simulink library "tvd"  (Simulink 8.1)
settings: Solver=ode1  StartTime=0.0  StopTime=Inf  FixedStep=0.001  RelTol=1e-3
PostLoadFcn:
  | , if any(exist('dsrtsu_mdlpostloadfcn', 'file') == [2, 3, 6]), try dsrtsu_mdlpostloadfcn('Execute', bdroot); catch fprintf('Error in PostLoadFcn (dsrtsu_mdlpostloadfcn) for model "%s":\n %s\n', bdroot, lasterr); end, end,
undefined symbols (not defined in the file or in its folder): C_TICK_TIME_S, KACC_MCLongAccelRollAvgInterval_s
libraries: hcu_lib x1
settings Model: DSRTSU_INTERNAL_RTI_VER=450  DSRTSU_INTERNAL_RTI_TYPE=rti1401  RTICANMMDATA=struct('GeneralSetupData',struct('modelroot','D:\Projects\ELN150201\Repositories\Taiwan\trunk\AdasDragon\software\sw_development\arch\app\acc','generalsettings',struct('filesettings',struct('destfolder',struct('Name','RTICANMM_FILES','Check',1),'buildfolder',struct('Name','.','Check',1),'AbsDestfolder',struct('Name','D:\Projects\ELN150201\Repositories\Taiwan\trunk\AdasDragon\software\sw_development\arch\app\acc\RTICANMM_FILES'),'AbsBuildfolder',struct('Name','D:\Projects\ELN150201\Repositories\Taiwan\trunk\AdasDragon\software\sw_development\arch\app\acc'))),'options',struct('addpaths',1,'rmpaths',1,'addtrcexclusion',logical(1),'cannavigator',struct('checkmonitoring',0),'show_usrtrc',0,'use_usrtrc',0),'advanced',struct('options',[1 1 1 1 1 1 1 1 1 1 1 1 1 1 1 1 1 1 1 1 1 1 1 1 1 1 1 1 1 1 1 1 1 1 1 1 1 1 1 1 1 1 1 1 1 1 1 1 1 1 1 1 1 1 1 1 1 1 1 1 1 1 1 1 1 1 1 1 1 1 1 1 1 1 1 1 1 1 1 1 1 1 1 1 1 1 1 1 1 1 1 1 1 1 1 1 1 1 1 1]),'MPSetup',{{}},'modelname','Copy_of_scc','block','Copy_of_scc'))  DSRTSU_INTERNAL_RTIFPGA=40  Creator=AT015411  LastModifiedBy=AT015086

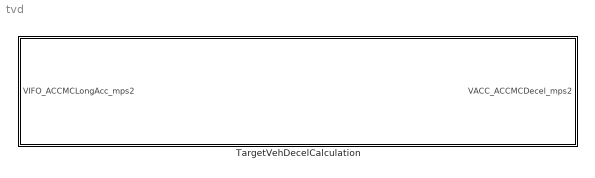
== system tvd ==
  TargetVehDecelCalculation : Subsystem

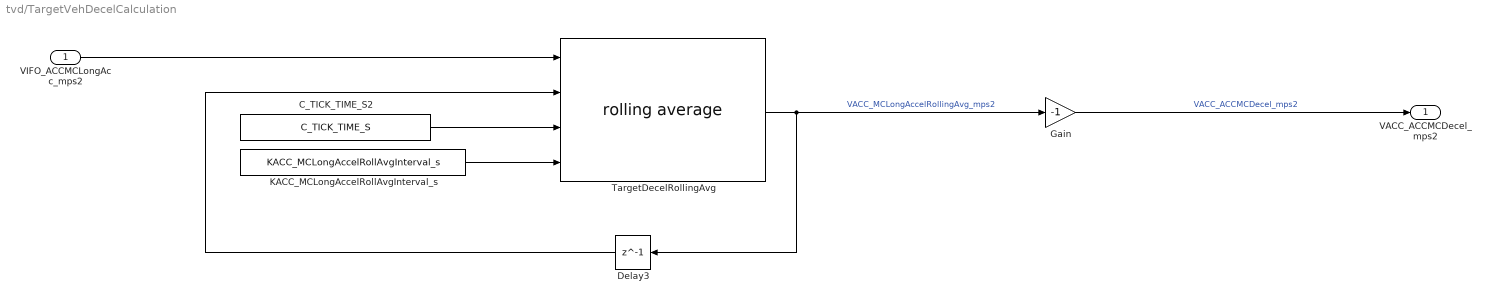
== system tvd/TargetVehDecelCalculation ==
  VIFO_ACCMCLongAcc_mps2 : Inport
  C_TICK_TIME_S2 : Constant  Value=C_TICK_TIME_S
  Delay3 : Delay  DelayLength=1
  Gain : Gain  Gain=-1
  KACC_MCLongAccelRollAvgInterval_s : Constant  Value=KACC_MCLongAccelRollAvgInterval_s
  TargetDecelRollingAvg : hcu_lib/rolling average
  VACC_ACCMCDecel_mps2 : Outport
  wires:
  Delay3/1 -> TargetDecelRollingAvg/2
  KACC_MCLongAccelRollAvgInterval_s/1 -> TargetDecelRollingAvg/4
  Gain/1 -> VACC_ACCMCDecel_mps2/1  "VACC_ACCMCDecel_mps2"
  C_TICK_TIME_S2/1 -> TargetDecelRollingAvg/3
  TargetDecelRollingAvg/1 -> Delay3/1, Gain/1  "VACC_MCLongAccelRollingAvg_mps2"
  VIFO_ACCMCLongAcc_mps2/1 -> TargetDecelRollingAvg/1
